simulink model "banana"  (R2015b)
settings: Solver=FixedStepDiscrete  StartTime=0.0  StopTime=Inf  FixedStep=0.01  RelTol=1e-3
undefined symbols (not defined in the file): Angular, Linear
libraries: robotlib x3, simulink x3
settings Model: Creator=The MathWorks, Inc.  LastModifiedBy=root
settings DataIOCC: SaveFormat=Array
settings OptimizationCC: OptimizeModelRefInitCode=on  LifeSpan=Inf  MaxStackSize=64
settings DebuggingCC: SolverPrmCheckMsg=warning
settings HardwareCC: ProdBitPerPointer=32  ProdLargestAtomicFloat=None  ProdIntDivRoundTo=Undefined  ProdEndianess=Unspecified  ProdWordSize=32  ProdHWDeviceType=Generic->Unspecified (assume 32-bit Generic)
settings RTWCC: SystemTargetFile=ert.tlc  TemplateMakefile=ert_default_tmf  Description=Embedded Coder  Toolchain=Catkin  TargetLang=C++
settings CodeAppCC: IgnoreCustomStorageClasses=off
settings ERTTargetCC: SupportVariableSizeSignals=on
settings ConfigComp: CovModelRefEnable=Off  CovSFcnEnable=off

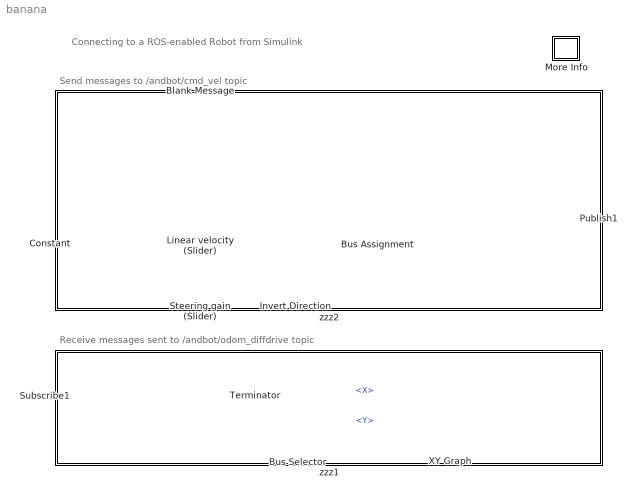
== system banana ==
  note: Receive messages sent to /andbot/odom_diffdrive topic
  note: Send messages to /andbot/cmd_vel topic
  note: Connecting to a ROS-enabled Robot from Simulink
  Blank Message : robotlib/Blank Message  SourceLibraryInfo=This block requires Robotics System Toolbox  messageType=geometry_msgs/Twist  SampleTime=inf
  Bus Assignment : BusAssignment  DialogController=Simulink.DDGSource_BusAssignment  AssignedSignals=Linear.X,Angular.Z
  Bus Selector : BusSelector  DialogController=Simulink.DDGSource_BusSelector  OutputSignals=Pose.Pose.Position.X,Pose.Pose.Position.Y
  Constant : Constant
  Invert Direction : Gain  Gain=-1
  Linear velocity (Slider) : simulink/Math Operations/Slider Gain  low=0  gain=0.5  high=2
  More Info : Subsystem
      settings: OpenFcn=showdemo(bdroot(gcb))
      mask Display: disp('?')
  Publish1 : robotlib/Publish  SourceLibraryInfo=This block requires Robotics System Toolbox  topicSource=Select from ROS network  topic=/andbot/cmd_vel  messageType=geometry_msgs/Twist  messageQueueLength=105
  Steering gain (Slider) : simulink/Math Operations/Slider Gain  low=-1  gain=0.3  high=1
  Subscribe1 : robotlib/Subscribe  SourceLibraryInfo=This block requires Robotics System Toolbox  topicSource=Select from ROS network  topic=/andbot/odom_diffdrive  messageType=nav_msgs/Odometry  sampleTime=-1  messageQueueLength=51
  Terminator : Terminator
  XY Graph : simulink/Sinks/XY Graph  xmin=-10  xmax=10  ymin=-10  ymax=10  st=-1
  zzz1 : Subsystem  TreatAsAtomicUnit=on
      settings: OpenFcn=% no-op
      mask Display: disp('')
  zzz2 : Subsystem  TreatAsAtomicUnit=on
      settings: OpenFcn=% no-op
      mask Display: disp('')
  wires:
  Bus Assignment/1 -> Publish1/1
  Blank Message/1 -> Bus Assignment/1
  Subscribe1/2 -> Bus Selector/1
  Bus Selector/1 -> XY Graph/1  "<X>"
  Bus Selector/2 -> XY Graph/2  "<Y>"
  Constant/1 -> Linear velocity (Slider)/1, Steering gain (Slider)/1
  Linear velocity (Slider)/1 -> Bus Assignment/2
  Steering gain (Slider)/1 -> Invert Direction/1
  Invert Direction/1 -> Bus Assignment/3
  Subscribe1/1 -> Terminator/1

== system banana/More Info ==

== system banana/zzz1 ==

== system banana/zzz2 ==
